simulink model "ampc_dc"  (Simulink 9.1)
settings: Solver=ode45  StartTime=0.0  StopTime=400  FixedStep=0.01  RelTol=1e-3
libraries: mpclib x1
settings Model: Creator=mulusoy  LastModifiedBy=Mehdi
settings DataIOCC: SaveFormat=StructureWithTime
settings OptimizationCC: DefaultParameterBehavior=Inlined  EnhancedBackFolding=on  PassReuseOutputArgsAs=Individual arguments
settings DebuggingCC: UnderspecifiedInitializationDetection=Simplified  MergeDetectMultiDrivingBlocksExec=error  ParameterTunabilityLossMsg=error  SFUnexpectedBacktrackingDiag=error  SFNoUnconditionalDefaultTransitionDiag=error
settings HardwareCC: ProdBitPerPointer=64  ProdLargestAtomicFloat=Float  ProdIntDivRoundTo=Zero  ProdEndianess=LittleEndian  ProdHWDeviceType=Specified
settings ModelReferenceCC: PropagateSignalLabelsOutOfModel=on
settings SFSimCC: MATLABDynamicMemAlloc=off
settings RTWCC: SystemTargetFile=ert.tlc  TemplateMakefile=ert_default_tmf  Description=Embedded Coder  GenerateReport=on  IncludeHyperlinkInReport=on  LaunchReport=on  GenerateTraceInfo=on  GenerateTraceReport=on  GenerateTraceReportSl=on  GenerateTraceReportSf=on  GenerateTraceReportEml=on
settings CodeAppCC: ForceParamTrailComments=on  IgnoreCustomStorageClasses=off  OperatorAnnotations=on  SimulinkDataObjDesc=on  SFDataObjDesc=on  InsertBlockDesc=on
settings ERTTargetCC: TargetLangStandard=C99 (ISO)  GenerateSampleERTMain=on  InlinedParameterPlacement=NonHierarchical  ERTCustomFileTemplate=example_file_process.tlc
settings ConfigComp: CovMetricSettings=dwe  CovHtmlReporting=off  CovSaveCumulativeToWorkspaceVar=off  CovSaveSingleToWorkspaceVar=off  CovExternalEMLEnable=on

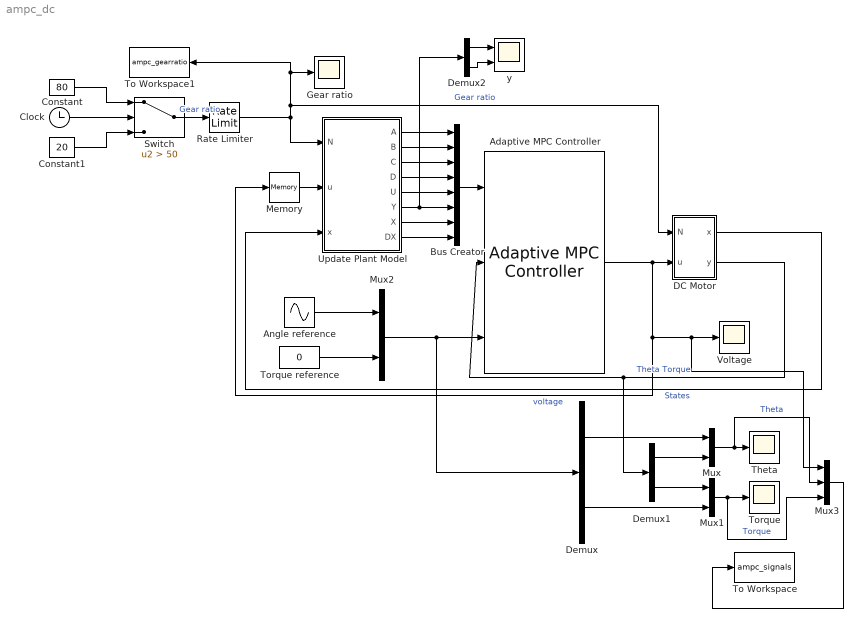
== system ampc_dc ==
  Adaptive MPC Controller : mpclib/Adaptive MPC Controller  SCDEnableBlockLinearizationSpecification=on  mpcobj=mpc1  x0=[]  updateMPCinCallerWorkspace=on  md_inport=off  mv_inport=off  cost_outport=off  return_sequence=off  return_qpstatus=off  return_state=off  state_inport=off  isltv_plant=off  lims_inport=off  cc_inport=off  ywt_inport=off  uwt_inport=off  duwt_inport=off  rhoeps_inport=off  uref_inport=off  BlockDataType=double  SampleTimeInherited=off  switch_inport=off
      settings: SourceProductName=Model Predictive Control Toolbox
  Angle reference : Sin  Amplitude=pi  Frequency=0.1  SampleTime=0
  Bus Creator : BusCreator  Inputs=8
  Clock : Clock
  Constant : Constant  Value=80
  Constant1 : Constant  Value=20
  DC Motor : Subsystem
  Demux : Demux  Outputs=2
  Demux1 : Demux  Outputs=2
  Demux2 : Demux  Outputs=2
  Gear ratio : Scope
  Memory : Memory
  Mux : Mux  Inputs=2
  Mux1 : Mux  Inputs=2
  Mux2 : Mux  Inputs=2
  Mux3 : Mux  Inputs=3
  Rate Limiter : RateLimiter  SampleTimeMode=inherited
  Switch : Switch  Criteria=u2 > Threshold  Threshold=50
  Theta : Scope
  To Workspace : ToWorkspace  VariableName=ampc_signals  SaveFormat=Timeseries  SampleTime=-1
  To Workspace1 : ToWorkspace  VariableName=ampc_gearratio  SaveFormat=Timeseries  SampleTime=0.1
  Torque : Scope
  Torque reference : Constant  Value=0
  Update Plant Model : MATLAB Function  TreatAsAtomicUnit=on
  Voltage : Scope
  y : Scope  NumInputPorts=2
  wires:
  Switch/1 -> Rate Limiter/1  "Gear ratio"
  Update Plant Model/1(A) -> Bus Creator/1
  Update Plant Model/2(B) -> Bus Creator/2
  Update Plant Model/3(C) -> Bus Creator/3
  Update Plant Model/4(D) -> Bus Creator/4
  Update Plant Model/5(U) -> Bus Creator/5
  Update Plant Model/6(Y) -> Demux2/1, Bus Creator/6
  Update Plant Model/7(X) -> Bus Creator/7
  Update Plant Model/8(DX) -> Bus Creator/8
  Bus Creator/1 -> Adaptive MPC Controller/1
  Adaptive MPC Controller/1 -> Mux3/1, Voltage/1, Memory/1, DC Motor/2(u)  "voltage"
  Mux2/1 -> Adaptive MPC Controller/3, Demux/1
  Demux/1 -> Mux/1
  Mux/1 -> Mux3/2, Theta/1  "Theta"
  Demux1/1 -> Mux/2
  Demux1/2 -> Mux1/1
  Demux/2 -> Mux1/2
  Mux1/1 -> Mux3/3, Torque/1  "Torque"
  DC Motor/2(y) -> Demux1/1, Adaptive MPC Controller/2  "Theta Torque"
  DC Motor/1(x) -> Update Plant Model/3(x)  "States"
  Memory/1 -> Update Plant Model/2(u)
  Angle reference/1 -> Mux2/1
  Torque reference/1 -> Mux2/2
  Constant/1 -> Switch/1
  Constant1/1 -> Switch/3
  Clock/1 -> Switch/2
  Mux3/1 -> To Workspace/1
  Demux2/1 -> y/1
  Demux2/2 -> y/2
  Rate Limiter/1 -> Update Plant Model/1(N), DC Motor/1(N), To Workspace1/1, Gear ratio/1  "Gear ratio"

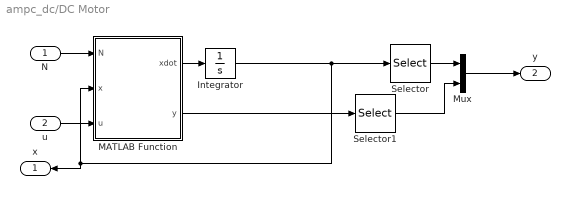
== system ampc_dc/DC Motor ==
  N : Inport
  u : Inport  Port=2
  Integrator : Integrator
  MATLAB Function : MATLAB Function  TreatAsAtomicUnit=on
  Mux : Mux  Inputs=2
  Selector : Selector  InputPortWidth=4  IndexOptions=Index vector (dialog)  Indices=[1]  OutputSizes=1
  Selector1 : Selector  InputPortWidth=1  IndexOptions=Index vector (dialog)  Indices=[1]  OutputSizes=1
  x : Outport
  y : Outport  Port=2
  wires:
  u/1 -> MATLAB Function/3(u)
  Integrator/1 -> Selector/1, x/1, MATLAB Function/2(x)
  MATLAB Function/1(xdot) -> Integrator/1
  N/1 -> MATLAB Function/1(N)
  Selector/1 -> Mux/1
  MATLAB Function/2(y) -> Selector1/1
  Mux/1 -> y/1
  Selector1/1 -> Mux/2

== matlab function Update Plant Model ==
  data: N input double; u input double; A output double size=[4,4]; x input double size=[4,1]; B output double size=[4,1]; C output double size=[2,4]; D output double size=[2,1]; U output double; Y output double size=[2,1]; X output double size=[4,1]; DX output double size=[4,1]
function [A,B,C,D,U,Y,X,DX] = fcn(N,u,x)
% Sample time
Ts = 0.1;

% Model parameters
Kt = 1280.2;  % Torsional rigidity
Km = 10;      % Motor constant
Jm = 0.5;     % Motor inertia
Jl = 50*Jm;   % Load inertia
Bm = 0.1;     % Rotor viscous friction
Bl = 25;      % Load viscous friction
R = 20;       % Armature resistance

Ac = [        0       1             0                0;
        -Kt/Jl  -Bl/Jl     Kt/(N*Jl)                0;
             0       0             0                1;
     Kt/(Jm*N)       0  -Kt/(Jm*N^2)  -(Bm+Km^2/R)/Jm];
Bc = [0; 0; 0; Km/(R*Jm)];
Cc = [  1  0       0  0;
      Kt  0   -Kt/N  0];
Dc = [0; 0];

% Generate discrete-time model
nx = size(Ac,1);
nu = size(Bc,2);
M = expm([[Ac Bc]*Ts; zeros(nu,nx+nu)]);
A = M(1:nx,1:nx);
B = M(1:nx,nx+1:nx+nu);
C = Cc;
D = Dc;

% Nominal conditions for discrete-time plant
X = x;
U = u;
Y = C*x + D*u;
DX = A*x+B*u-x;

== matlab function DC Motor/MATLAB Function ==
  data: N input double; x input double size=[4,1]; u input double; xdot output double size=[4,1]; y output double
function [xdot,y] = fcn(N,x,u)

% Model parameters
Kt = 1280.2;  % Torsional rigidity
Km = 10;      % Motor constant
Jm = 0.5;     % Motor inertia
Jl = 50*Jm;   % Load inertia
Bm = 0.1;     % Rotor viscous friction
Bl = 25;      % Load viscous friction
R = 20;       % Armature resistance

A = [        0       1             0                0;
        -Kt/Jl  -Bl/Jl     Kt/(N*Jl)                0;
             0       0             0                1;
     Kt/(Jm*N)       0  -Kt/(Jm*N^2)  -(Bm+Km^2/R)/Jm];
B = [0; 0; 0; Km/(R*Jm)];

C = [Kt  0   -Kt/N  0];
xdot = A*x + B*u;
y = C*x;
